simulink model "dVOC_control_demo_fault_2023b_Psensitivity"  (R2023b)
settings: Solver=ode23tb  StartTime=0.0  StopTime=Tend  RelTol=1e-3
values from neighbouring files (symbols this model uses):
  alpha = 1e-1*V_m^2    [dVOC_control_Psensitivity.m]    (also in dVOC_control_demo.m)
  C_4 = 0.1670*C_b    (= 1.00487241952e-06)    [dVOC_control_Psensitivity.m]    (also in dVOC_control_demo.m)
  C_8 = 0.2275*C_b    (= 1.36891302659e-06)    [dVOC_control_Psensitivity.m]    (also in dVOC_control_demo.m)
  C_dc = 0.008*(n)    (= 1.6)    [dVOC_control_Psensitivity.m]    (also in dVOC_control_demo.m)
  C_f = n*300*10^-6    (= 0.06)    [dVOC_control_Psensitivity.m]    (also in dVOC_control_demo.m)
  dp = P_delta((i_loc-1)*10+i_p)    [dVOC_control_Psensitivity.m]
  droop_percentage = 1    [dVOC_control_Psensitivity.m]    (also in dVOC_control_demo.m)
  eta = m_p*V_m^2    [dVOC_control_Psensitivity.m]    (also in dVOC_control_demo.m)
  i_ll = -1.15*(S_b/Vdc_n)-i_loss_dc    [dVOC_control_Psensitivity.m]    (also in dVOC_control_demo.m)
  i_ul = 1.15*(S_b/Vdc_n)+i_loss_dc    [dVOC_control_Psensitivity.m]    (also in dVOC_control_demo.m)
  k_dc = eta_1/(Vdc_n*m_p)    [dVOC_control_Psensitivity.m]    (also in dVOC_control_demo.m)
  K_p = (1/Vdc_n)    [dVOC_control_Psensitivity.m]    (also in dVOC_control_demo.m)
  K_r = 1/R_dc    [dVOC_control_Psensitivity.m]    (also in dVOC_control_demo.m)
  Kff_i = 1    [dVOC_control_Psensitivity.m]    (also in dVOC_control_demo.m)
  Kff_v = 1    [dVOC_control_Psensitivity.m]    (also in dVOC_control_demo.m)
  Ki_i = (1/n)*1.19    (= 0.00595)    [dVOC_control_Psensitivity.m]    (also in dVOC_control_demo.m)
  Ki_v = (n)*1.161022    (= 232.2044)    [dVOC_control_Psensitivity.m]    (also in dVOC_control_demo.m)
  Kp_i = 0.738891    [dVOC_control_Psensitivity.m]    (also in dVOC_control_demo.m)
  Kp_v = 0.52    [dVOC_control_Psensitivity.m]    (also in dVOC_control_demo.m)
  L1_pu = 1*0.0186/m    (= 0.000186)    [dVOC_control_Psensitivity.m]    (also in dVOC_control_demo.m)
  L_45 = L_lines(2)    [dVOC_control_Psensitivity.m]    (also in dVOC_control_demo.m)
  L_89 = L_lines(8)    [dVOC_control_Psensitivity.m]    (also in dVOC_control_demo.m)
  L_94 = L_lines(9)    [dVOC_control_Psensitivity.m]    (also in dVOC_control_demo.m)
  L_f = (1/n)*200*10^-6    (= 1e-06)    [dVOC_control_Psensitivity.m]    (also in dVOC_control_demo.m)
  n = 200    [dVOC_control_Psensitivity.m]    (also in dVOC_control_demo.m)
  pl = S_b*ps    (= 75000000)    [dVOC_control_Psensitivity.m]    (also in dVOC_control_demo.m)
  ps = base/3    (= 0.75)    [dVOC_control_Psensitivity.m]    (also in dVOC_control_demo.m)
  qs = [0;0]    [dVOC_control_Psensitivity.m]    (also in dVOC_control_demo.m)
  R1_pu = 1*0.00734/m    (= 7.34e-05)    [dVOC_control_Psensitivity.m]    (also in dVOC_control_demo.m)
  R_45 = R_lines(2)    [dVOC_control_Psensitivity.m]    (also in dVOC_control_demo.m)
  R_89 = R_lines(8)    [dVOC_control_Psensitivity.m]    (also in dVOC_control_demo.m)
  R_94 = R_lines(9)    [dVOC_control_Psensitivity.m]    (also in dVOC_control_demo.m)
  R_dc = (Vdc_n/(0.05*(S_b)/Vdc_n))    [dVOC_control_Psensitivity.m]    (also in dVOC_control_demo.m)
  R_f = 0.001/n    (= 5e-06)    [dVOC_control_Psensitivity.m]    (also in dVOC_control_demo.m)
  S_b = 100*(10^6)    (= 100000000)    [dVOC_control_Psensitivity.m]    (also in dVOC_control_demo.m)
  S_bt = S_b    (= 100000000)    [dVOC_control_Psensitivity.m]    (also in dVOC_control_demo.m)
  t_disturbance = linspace(0.01,0.2,10)    [dVOC_control_Psensitivity.m]    (also in dVOC_control_demo.m; data_post_process_ExtendSmooth.m = 5+linspace(0.01,0.2,n_period); data_post_process_ExtendSmooth_Psensitivity.m = 5+linspace(0.0,0.0,n_period))
  T_en = T_load(1)-0.5    [dVOC_control_Psensitivity.m]    (also in dVOC_control_demo.m)
  T_load = [5 5]    [dVOC_control_Psensitivity.m]    (also in dVOC_control_demo.m = [5 5.2])
  T_load1 = [T_load(1)-dt_load(1), T_load(1)]    [dVOC_control_Psensitivity.m]    (also in dVOC_control_demo.m = [T_load(1), T_load(1) + dt_load(1)])
  T_load2 = [T_load(1)-dt_load(2), T_load(1)]    [dVOC_control_Psensitivity.m]    (also in dVOC_control_demo.m = [T_load(1), T_load(1) + dt_load(2)])
  T_loss = Tend    (= 8)    [dVOC_control_Psensitivity.m]    (also in dVOC_control_demo.m)
  T_s = 3.125e-4/4    (= 7.8125e-05)    [dVOC_control_Psensitivity.m]    (also in dVOC_control_demo.m)
  tau_dc = 0.05    [dVOC_control_Psensitivity.m]    (also in dVOC_control_demo.m)
  tau_g = 5    [dVOC_control_Psensitivity.m]    (also in dVOC_control_demo.m)
  V1_rms = 1000    [dVOC_control_Psensitivity.m]    (also in dVOC_control_demo.m)
  V2_rms = 13800    [dVOC_control_Psensitivity.m]    (also in dVOC_control_demo.m)
  V_m = sqrt(2/3)*V1_rms    [dVOC_control_Psensitivity.m]    (also in dVOC_control_demo.m)
  Vdc_n = 3*V_m    [dVOC_control_Psensitivity.m]    (also in dVOC_control_demo.m)
  w_b = 2*pi*f_b    (= 314.159265359)    [dVOC_control_Psensitivity.m]    (also in dVOC_control_demo.m)
  w_f = 2*pi*5    (= 31.4159265359)    [dVOC_control_Psensitivity.m]    (also in dVOC_control_demo.m)
undefined symbols (not defined in the file or in its folder): D1, Delta, i_dc, i_t
libraries: eePMU x12, simulink_extras x9, spsabctoAlphaBetaZeroLib x9, spsSeriesRLCBranchLib x8, spsVoltageMeasurementLib x7, spsThreePhaseVIMeasurementLib x6, spsCurrentMeasurementLib x6, spsabctodq0Lib x6, spsGroundLib x5, spsThreePhaseParallelRLCLoadLib x3, spsThreePhaseBreakerLib x3, cstblocks x3
(part 2 of 2)

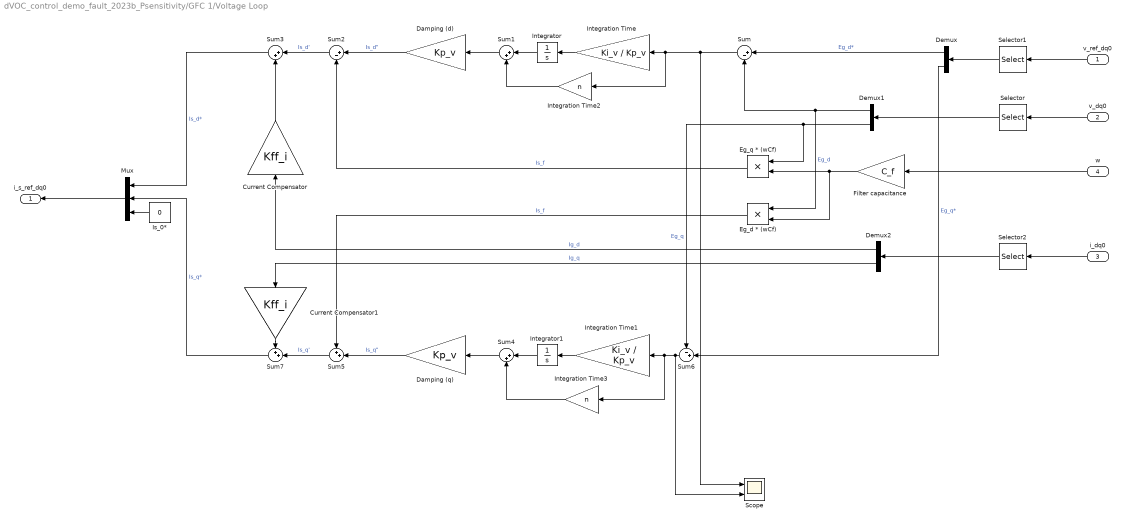
== system dVOC_control_demo_fault_2023b_Psensitivity/GFC 1/Voltage Loop ==
  v_ref_dq0 : Inport
  v_dq0 : Inport  Port=2
  i_dq0 : Inport  Port=3
  w : Inport  Port=4
  Current Compensator : Gain  Gain=Kff_i
  Current Compensator1 : Gain  Gain=Kff_i
  Damping (d) : Gain  Gain=Kp_v
  Damping (q) : Gain  Gain=Kp_v
  Demux : Demux  Outputs=2
  Demux1 : Demux  Outputs=2
  Demux2 : Demux  Outputs=2
  Eg_d * (wCf) : Product  RndMeth=Zero
  "Eg_q * (wCf) " : Product  RndMeth=Zero
  Filter capacitance : Gain  Gain=C_f
  Integration Time : Gain  Gain=Ki_v / Kp_v
  Integration Time1 : Gain  Gain=Ki_v / Kp_v
  Integration Time2 : Gain  Gain=n
  Integration Time3 : Gain  Gain=n
  Integrator : Integrator
  Integrator1 : Integrator
  Is_0* : Constant  Value=0
  Mux : Mux  Inputs=3
  Scope : Scope  NumInputPorts=2
  Selector : Selector  InputPortWidth=3  IndexOptions=Index vector (dialog)  Indices=[1 2]  OutputSizes=1
  Selector1 : Selector  InputPortWidth=3  IndexOptions=Index vector (dialog)  Indices=[1 2]  OutputSizes=1
  Selector2 : Selector  InputPortWidth=3  IndexOptions=Index vector (dialog)  Indices=[1 2]  OutputSizes=1
  Sum : Sum  Inputs=|+-
  Sum1 : Sum  Inputs=|++
  Sum2 : Sum  Inputs=|+-
  Sum3 : Sum  Inputs=|++
  Sum4 : Sum  Inputs=|++
  Sum5 : Sum  Inputs=++|
  Sum6 : Sum  Inputs=-+|
  Sum7 : Sum  Inputs=++|
  i_s_ref_dq0 : Outport  VectorParamsAs1DForOutWhenUnconnected=off
  wires:
  Is_0*/1 -> Mux/3
  w/1 -> Filter capacitance/1
  Integration Time1/1 -> Integrator1/1
  Integrator1/1 -> Sum4/1
  Demux/2 -> Sum6/2  "Eg_q*"
  v_ref_dq0/1 -> Selector1/1
  Eg_d * (wCf)/1 -> Sum5/1  "Is_f"
  Sum7/1 -> Mux/2  "Is_q*"
  Demux2/2 -> Current Compensator1/1  "Ig_q"
  Demux/1 -> Sum/1  "Eg_d*"
  Sum6/1 -> Scope/2, Integration Time3/1, Integration Time1/1
  Demux2/1 -> Current Compensator/1  "Ig_d"
  Sum2/1 -> Sum3/1  "Is_d'"
  Current Compensator/1 -> Sum3/2
  Demux1/1 -> Eg_d * (wCf)/1, Sum/2  "Eg_d"
  Current Compensator1/1 -> Sum7/1
  "Eg_q * (wCf) "/1 -> Sum2/2  "Is_f"
  Demux1/2 -> "Eg_q * (wCf) "/1, Sum6/1  "Eg_q"
  Filter capacitance/1 -> "Eg_q * (wCf) "/2, Eg_d * (wCf)/2
  Damping (d)/1 -> Sum2/1  "Is_d\""
  i_dq0/1 -> Selector2/1
  Sum5/1 -> Sum7/2  "Is_q'"
  Sum1/1 -> Damping (d)/1
  Integrator/1 -> Sum1/1
  Integration Time/1 -> Integrator/1
  Sum4/1 -> Damping (q)/1
  Sum3/1 -> Mux/1  "Is_d*"
  v_dq0/1 -> Selector/1
  Damping (q)/1 -> Sum5/2  "Is_q\""
  Selector/1 -> Demux1/1
  Selector1/1 -> Demux/1
  Selector2/1 -> Demux2/1
  Mux/1 -> i_s_ref_dq0/1
  Sum/1 -> Scope/1, Integration Time/1, Integration Time2/1
  Integration Time2/1 -> Sum1/2
  Integration Time3/1 -> Sum4/2

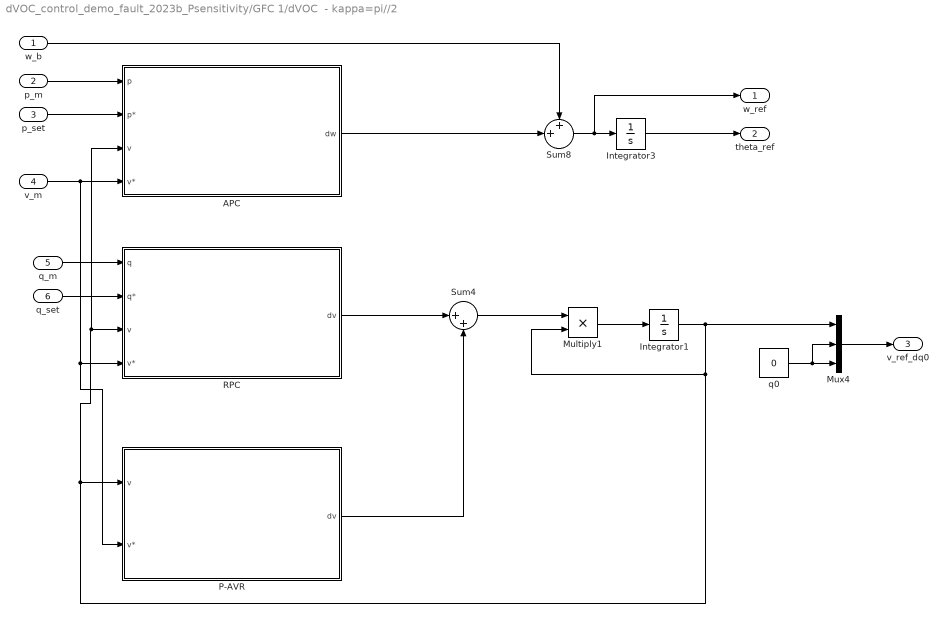
== system dVOC_control_demo_fault_2023b_Psensitivity/GFC 1/dVOC  - kappa=pi//2 ==
  w_b : Inport
  p_m : Inport  Port=2
  p_set : Inport  Port=3
  v_m : Inport  Port=4
  q_m : Inport  Port=5
  q_set : Inport  Port=6
  APC : Subsystem
  Integrator1 : Integrator  InitialCondition=V_m
  Integrator3 : Integrator
  Multiply1 : Product
  Mux4 : Mux  Inputs=3
  P-AVR : Subsystem
  RPC : Subsystem
  Sum4 : Sum  Inputs=|++
  Sum8 : Sum  Inputs=++|
  q0 : Constant  Value=0
  w_ref : Outport  VectorParamsAs1DForOutWhenUnconnected=off
  theta_ref : Outport  Port=2  VectorParamsAs1DForOutWhenUnconnected=off
  v_ref_dq0 : Outport  Port=3  VectorParamsAs1DForOutWhenUnconnected=off
  wires:
  Mux4/1 -> v_ref_dq0/1
  q0/1 -> Mux4/3, Mux4/2
  Sum8/1 -> Integrator3/1, w_ref/1
  w_b/1 -> Sum8/1
  Integrator3/1 -> theta_ref/1
  p_m/1 -> APC/1(p)
  p_set/1 -> APC/2(p*)
  APC/1(dw) -> Sum8/2
  q_m/1 -> RPC/1(q)
  q_set/1 -> RPC/2(q*)
  Integrator1/1 -> Multiply1/2, APC/3(v), RPC/3(v), P-AVR/1(v), Mux4/1
  Sum4/1 -> Multiply1/1
  v_m/1 -> P-AVR/2(v*), RPC/4(v*), APC/4(v*)
  P-AVR/1(dv) -> Sum4/2
  Multiply1/1 -> Integrator1/1
  RPC/1(dv) -> Sum4/1

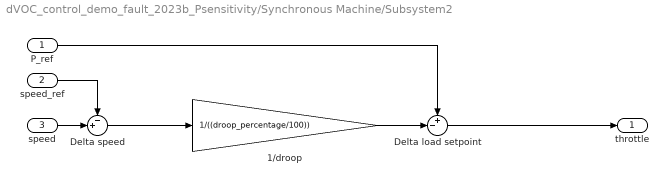
== system dVOC_control_demo_fault_2023b_Psensitivity/Synchronous Machine/Subsystem2 ==
  P_ref : Inport
  speed_ref : Inport  Port=2
  speed : Inport  Port=3
  1/droop : Gain  Gain=1/((droop_percentage/100))
  Delta load setpoint : Sum  Inputs=+-|
  Delta speed : Sum  Inputs=-+|
  throttle : Outport  VectorParamsAs1DForOutWhenUnconnected=off
  wires:
  speed/1 -> Delta speed/2
  1/droop/1 -> Delta load setpoint/2
  Delta speed/1 -> 1/droop/1
  speed_ref/1 -> Delta speed/1
  P_ref/1 -> Delta load setpoint/1
  Delta load setpoint/1 -> throttle/1

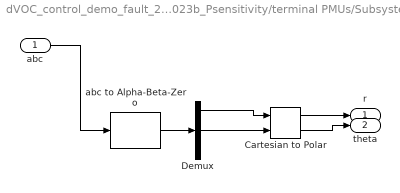
== system dVOC_control_demo_fault_2023b_Psensitivity/terminal PMUs/Subsystem1 ==
  abc : Inport
  Cartesian to Polar : simulink_extras/Transformations/Cartesian to Polar
  Demux : Demux  Outputs=3
  abc to Alpha-Beta-Zero : spsabctoAlphaBetaZeroLib/abc to Alpha-Beta-Zero
  r : Outport
  theta : Outport  Port=2
  wires:
  Demux/1 -> Cartesian to Polar/1
  abc to Alpha-Beta-Zero/1 -> Demux/1
  Demux/2 -> Cartesian to Polar/2
  abc/1 -> abc to Alpha-Beta-Zero/1
  Cartesian to Polar/1 -> r/1
  Cartesian to Polar/2 -> theta/1

== system dVOC_control_demo_fault_2023b_Psensitivity/terminal PMUs/Subsystem2 ==
  abc : Inport
  Cartesian to Polar : simulink_extras/Transformations/Cartesian to Polar
  Demux : Demux  Outputs=3
  abc to Alpha-Beta-Zero : spsabctoAlphaBetaZeroLib/abc to Alpha-Beta-Zero
  r : Outport
  theta : Outport  Port=2
  wires:
  Demux/1 -> Cartesian to Polar/1
  abc to Alpha-Beta-Zero/1 -> Demux/1
  Demux/2 -> Cartesian to Polar/2
  abc/1 -> abc to Alpha-Beta-Zero/1
  Cartesian to Polar/1 -> r/1
  Cartesian to Polar/2 -> theta/1

== system dVOC_control_demo_fault_2023b_Psensitivity/terminal PMUs/Subsystem3 ==
  abc : Inport
  Cartesian to Polar : simulink_extras/Transformations/Cartesian to Polar
  Demux : Demux  Outputs=3
  abc to Alpha-Beta-Zero : spsabctoAlphaBetaZeroLib/abc to Alpha-Beta-Zero
  r : Outport
  theta : Outport  Port=2
  wires:
  Demux/1 -> Cartesian to Polar/1
  abc to Alpha-Beta-Zero/1 -> Demux/1
  Demux/2 -> Cartesian to Polar/2
  abc/1 -> abc to Alpha-Beta-Zero/1
  Cartesian to Polar/1 -> r/1
  Cartesian to Polar/2 -> theta/1

== system dVOC_control_demo_fault_2023b_Psensitivity/terminal PMUs/Subsystem4 ==
  abc : Inport
  Cartesian to Polar : simulink_extras/Transformations/Cartesian to Polar
  Demux : Demux  Outputs=3
  abc to Alpha-Beta-Zero : spsabctoAlphaBetaZeroLib/abc to Alpha-Beta-Zero
  r : Outport
  theta : Outport  Port=2
  wires:
  Demux/1 -> Cartesian to Polar/1
  abc to Alpha-Beta-Zero/1 -> Demux/1
  Demux/2 -> Cartesian to Polar/2
  abc/1 -> abc to Alpha-Beta-Zero/1
  Cartesian to Polar/1 -> r/1
  Cartesian to Polar/2 -> theta/1

== system dVOC_control_demo_fault_2023b_Psensitivity/terminal PMUs/Subsystem5 ==
  abc : Inport
  Cartesian to Polar : simulink_extras/Transformations/Cartesian to Polar
  Demux : Demux  Outputs=3
  abc to Alpha-Beta-Zero : spsabctoAlphaBetaZeroLib/abc to Alpha-Beta-Zero
  r : Outport
  theta : Outport  Port=2
  wires:
  Demux/1 -> Cartesian to Polar/1
  abc to Alpha-Beta-Zero/1 -> Demux/1
  Demux/2 -> Cartesian to Polar/2
  abc/1 -> abc to Alpha-Beta-Zero/1
  Cartesian to Polar/1 -> r/1
  Cartesian to Polar/2 -> theta/1

== system dVOC_control_demo_fault_2023b_Psensitivity/terminal PMUs/Subsystem6 ==
  abc : Inport
  Cartesian to Polar : simulink_extras/Transformations/Cartesian to Polar
  Demux : Demux  Outputs=3
  abc to Alpha-Beta-Zero : spsabctoAlphaBetaZeroLib/abc to Alpha-Beta-Zero
  r : Outport
  theta : Outport  Port=2
  wires:
  Demux/1 -> Cartesian to Polar/1
  abc to Alpha-Beta-Zero/1 -> Demux/1
  Demux/2 -> Cartesian to Polar/2
  abc/1 -> abc to Alpha-Beta-Zero/1
  Cartesian to Polar/1 -> r/1
  Cartesian to Polar/2 -> theta/1

== system dVOC_control_demo_fault_2023b_Psensitivity/terminal PMUs/Subsystem7 ==
  abc : Inport
  Cartesian to Polar : simulink_extras/Transformations/Cartesian to Polar
  Demux : Demux  Outputs=3
  abc to Alpha-Beta-Zero : spsabctoAlphaBetaZeroLib/abc to Alpha-Beta-Zero
  r : Outport
  theta : Outport  Port=2
  wires:
  Demux/1 -> Cartesian to Polar/1
  abc to Alpha-Beta-Zero/1 -> Demux/1
  Demux/2 -> Cartesian to Polar/2
  abc/1 -> abc to Alpha-Beta-Zero/1
  Cartesian to Polar/1 -> r/1
  Cartesian to Polar/2 -> theta/1

== system dVOC_control_demo_fault_2023b_Psensitivity/terminal PMUs/Subsystem8 ==
  abc : Inport
  Cartesian to Polar : simulink_extras/Transformations/Cartesian to Polar
  Demux : Demux  Outputs=3
  abc to Alpha-Beta-Zero : spsabctoAlphaBetaZeroLib/abc to Alpha-Beta-Zero
  r : Outport
  theta : Outport  Port=2
  wires:
  Demux/1 -> Cartesian to Polar/1
  abc to Alpha-Beta-Zero/1 -> Demux/1
  Demux/2 -> Cartesian to Polar/2
  abc/1 -> abc to Alpha-Beta-Zero/1
  Cartesian to Polar/1 -> r/1
  Cartesian to Polar/2 -> theta/1

== system dVOC_control_demo_fault_2023b_Psensitivity/terminal PMUs/Subsystem9 ==
  abc : Inport
  Cartesian to Polar : simulink_extras/Transformations/Cartesian to Polar
  Demux : Demux  Outputs=3
  abc to Alpha-Beta-Zero : spsabctoAlphaBetaZeroLib/abc to Alpha-Beta-Zero
  r : Outport
  theta : Outport  Port=2
  wires:
  Demux/1 -> Cartesian to Polar/1
  abc to Alpha-Beta-Zero/1 -> Demux/1
  Demux/2 -> Cartesian to Polar/2
  abc/1 -> abc to Alpha-Beta-Zero/1
  Cartesian to Polar/1 -> r/1
  Cartesian to Polar/2 -> theta/1

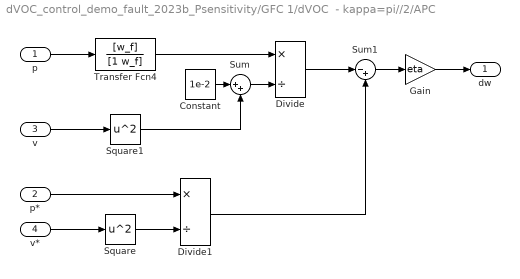
== system dVOC_control_demo_fault_2023b_Psensitivity/GFC 1/dVOC  - kappa=pi//2/APC ==
  p : Inport
  p* : Inport  Port=2
  v : Inport  Port=3
  v* : Inport  Port=4
  Constant : Constant  Value=1e-2
  Divide : Product  Inputs=*/
  Divide1 : Product  Inputs=*/
  Gain : Gain  Gain=eta
  Square : Math  Operator=square  SignedPower=on
  Square1 : Math  Operator=square  SignedPower=on
  Sum : Sum  Inputs=|++
  Sum1 : Sum  Inputs=|-+
  Transfer Fcn4 : TransferFcn  Numerator=[w_f]  Denominator=[1 w_f]
  dw : Outport  VectorParamsAs1DForOutWhenUnconnected=off
  wires:
  p/1 -> Transfer Fcn4/1
  p*/1 -> Divide1/1
  Transfer Fcn4/1 -> Divide/1
  v/1 -> Square1/1
  Constant/1 -> Sum/1
  Sum/1 -> Divide/2
  v*/1 -> Square/1
  Square/1 -> Divide1/2
  Square1/1 -> Sum/2
  Divide/1 -> Sum1/1
  Divide1/1 -> Sum1/2
  Sum1/1 -> Gain/1
  Gain/1 -> dw/1

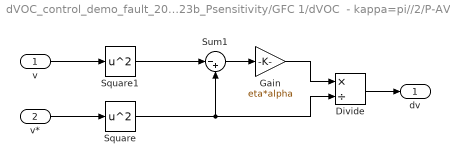
== system dVOC_control_demo_fault_2023b_Psensitivity/GFC 1/dVOC  - kappa=pi//2/P-AVR ==
  v : Inport
  v* : Inport  Port=2
  Divide : Product  Inputs=*/
  Gain : Gain  Gain=eta*alpha
  Square : Math  Operator=square  SignedPower=on
  Square1 : Math  Operator=square  SignedPower=on
  Sum1 : Sum  Inputs=|-+
  dv : Outport  VectorParamsAs1DForOutWhenUnconnected=off
  wires:
  v/1 -> Square1/1
  v*/1 -> Square/1
  Square/1 -> Sum1/2, Divide/2
  Sum1/1 -> Gain/1
  Square1/1 -> Sum1/1
  Gain/1 -> Divide/1
  Divide/1 -> dv/1

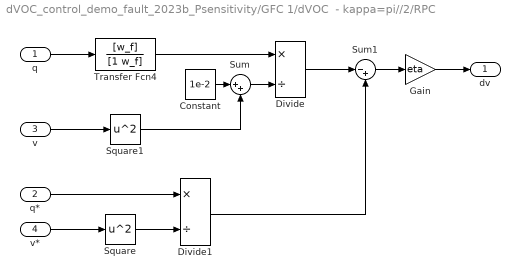
== system dVOC_control_demo_fault_2023b_Psensitivity/GFC 1/dVOC  - kappa=pi//2/RPC ==
  q : Inport
  q* : Inport  Port=2
  v : Inport  Port=3
  v* : Inport  Port=4
  Constant : Constant  Value=1e-2
  Divide : Product  Inputs=*/
  Divide1 : Product  Inputs=*/
  Gain : Gain  Gain=eta
  Square : Math  Operator=square  SignedPower=on
  Square1 : Math  Operator=square  SignedPower=on
  Sum : Sum  Inputs=|++
  Sum1 : Sum  Inputs=|-+
  Transfer Fcn4 : TransferFcn  Numerator=[w_f]  Denominator=[1 w_f]
  dv : Outport  VectorParamsAs1DForOutWhenUnconnected=off
  wires:
  q/1 -> Transfer Fcn4/1
  q*/1 -> Divide1/1
  Transfer Fcn4/1 -> Divide/1
  Constant/1 -> Sum/1
  Sum/1 -> Divide/2
  v*/1 -> Square/1
  Square/1 -> Divide1/2
  Square1/1 -> Sum/2
  Divide/1 -> Sum1/1
  Divide1/1 -> Sum1/2
  Sum1/1 -> Gain/1
  Gain/1 -> dv/1
  v/1 -> Square1/1
